simulink model "cIPC_leakyIntegrator"  (R2022a)
settings: Solver=FixedStepDiscrete  StartTime=0.0  StopTime=TMax  FixedStep=DT  RelTol=1e-3
undefined symbols (not defined in the file): DiscIntNeverNeededParam, dMdTheta, DT, K_T, Ki, optimal_azimuth_offset_rad
libraries: cstblocks x2
settings Model: Creator=jhummel  LastModifiedBy=jhummel

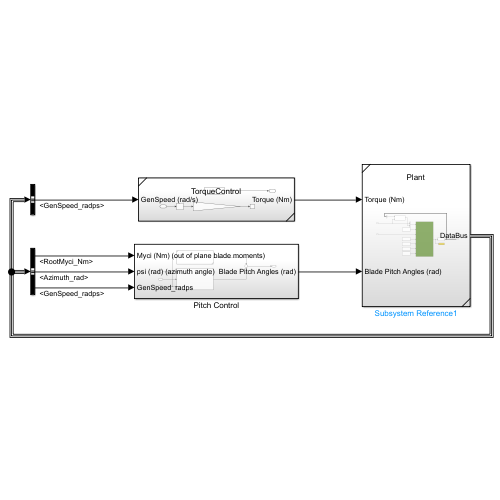
[thumbnail: Simulink's stored preview of the top-level diagram]
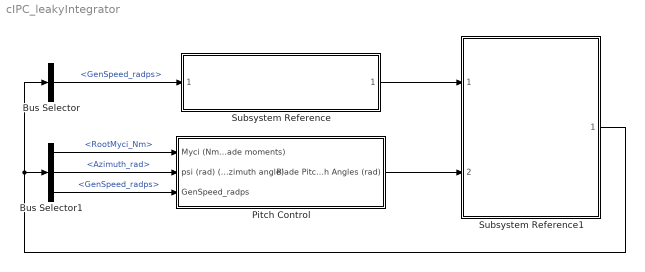
== system cIPC_leakyIntegrator ==
  Bus Selector : BusSelector  OutputSignals=GenSpeed_radps
  Bus Selector1 : BusSelector  OutputSignals=RootMyci_Nm,Azimuth_rad,GenSpeed_radps
  Pitch Control : Subsystem
  Subsystem Reference : Subsystem  ReferencedSubsystem=TorqueControl
  Subsystem Reference1 : Subsystem  ReferencedSubsystem=Plant
  wires:
  Bus Selector/1 -> Subsystem Reference/1  "<GenSpeed_radps>"
  Bus Selector1/1 -> Pitch Control/1(Myci (Nm) (out of plane blade moments))  "<RootMyci_Nm>"
  Bus Selector1/2 -> Pitch Control/2(psi (rad) (azimuth angle))  "<Azimuth_rad>"
  Bus Selector1/3 -> Pitch Control/3(GenSpeed_radps)  "<GenSpeed_radps>"
  Subsystem Reference1/1 -> Bus Selector/1, Bus Selector1/1
  Pitch Control/1(Blade Pitch Angles (rad)) -> Subsystem Reference1/2
  Subsystem Reference/1 -> Subsystem Reference1/1

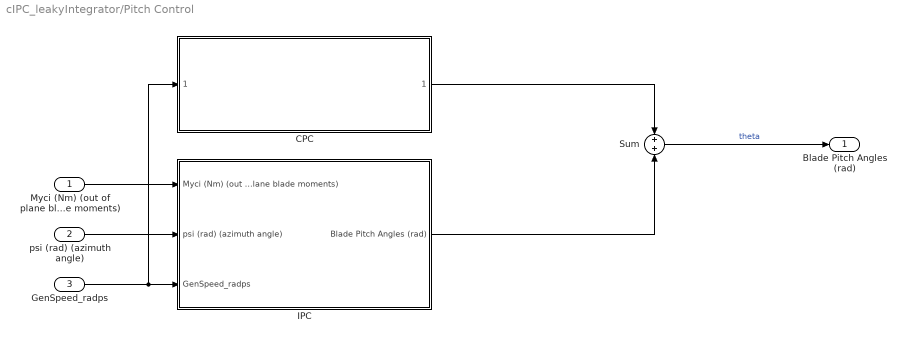
== system cIPC_leakyIntegrator/Pitch Control ==
  Myci (Nm) (out of plane blade moments) : Inport
  psi (rad) (azimuth angle) : Inport  Port=2
  GenSpeed_radps : Inport  Port=3
  CPC : Subsystem  ReferencedSubsystem=CollectivePitchControl
  IPC : Subsystem
  Sum : Sum  Inputs=+|+
  Blade Pitch Angles (rad) : Outport
  wires:
  Myci (Nm) (out of plane blade moments)/1 -> IPC/1(Myci (Nm) (out of plane blade moments))
  psi (rad) (azimuth angle)/1 -> IPC/2(psi (rad) (azimuth angle))
  GenSpeed_radps/1 -> CPC/1, IPC/3(GenSpeed_radps)
  Sum/1 -> Blade Pitch Angles (rad)/1  "theta"
  IPC/1(Blade Pitch Angles (rad)) -> Sum/2
  CPC/1 -> Sum/1

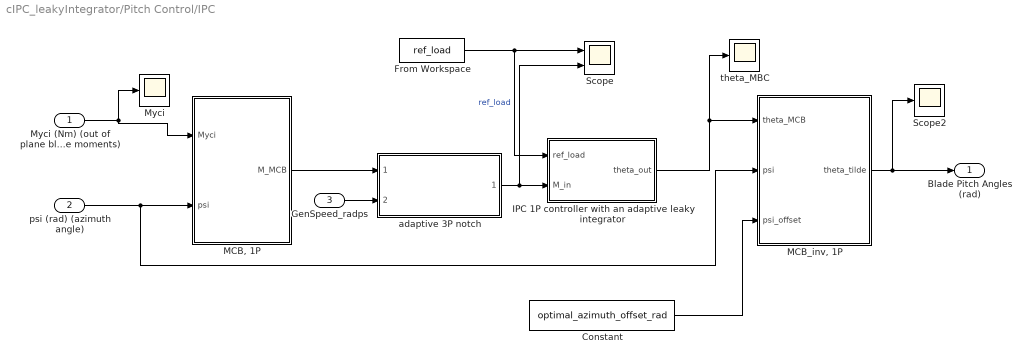
== system cIPC_leakyIntegrator/Pitch Control/IPC ==
  Myci (Nm) (out of plane blade moments) : Inport
  psi (rad) (azimuth angle) : Inport  Port=2
  GenSpeed_radps : Inport  Port=3
  Constant : Constant  Value=optimal_azimuth_offset_rad
  From Workspace : FromWorkspace  VariableName=ref_load  SampleTime=DT
  IPC 1P controller with an adaptive leaky integrator : Subsystem
  "MCB, 1P" : MATLAB Function  TreatAsAtomicUnit=on
  "MCB_inv, 1P" : MATLAB Function  TreatAsAtomicUnit=on
  Myci : Scope
  Scope : Scope  NumInputPorts=2
  Scope2 : Scope
  adaptive 3P notch : Subsystem  ReferencedSubsystem=LoadFilter
  theta_MBC : Scope
  Blade Pitch Angles (rad) : Outport
  wires:
  IPC 1P controller with an adaptive leaky integrator/1(theta_out) -> theta_MBC/1, "MCB_inv, 1P"/1(theta_MCB)
  "MCB_inv, 1P"/1(theta_tilde) -> Blade Pitch Angles (rad)/1, Scope2/1
  Myci (Nm) (out of plane blade moments)/1 -> Myci/1, "MCB, 1P"/1(Myci)
  Constant/1 -> "MCB_inv, 1P"/3(psi_offset)
  psi (rad) (azimuth angle)/1 -> "MCB_inv, 1P"/2(psi), "MCB, 1P"/2(psi)
  adaptive 3P notch/1 -> Scope/2, IPC 1P controller with an adaptive leaky integrator/2(M_in)
  GenSpeed_radps/1 -> adaptive 3P notch/2
  "MCB, 1P"/1(M_MCB) -> adaptive 3P notch/1
  From Workspace/1 -> Scope/1, IPC 1P controller with an adaptive leaky integrator/1(ref_load)  "ref_load"

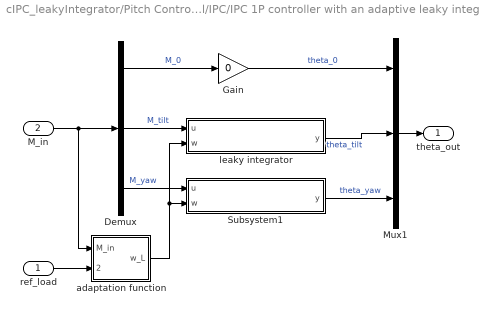
== system cIPC_leakyIntegrator/Pitch Control/IPC/IPC 1P controller with an adaptive leaky integrator ==
  ref_load : Inport
  M_in : Inport  Port=2
  Demux : Demux  Outputs=3
  Gain : Gain  Gain=0
  Mux1 : Mux  Inputs=3
  Subsystem1 : Subsystem
  adaptation function : Subsystem
  leaky integrator : Subsystem
  theta_out : Outport
  wires:
  Gain/1 -> Mux1/1  "theta_0"
  leaky integrator/1(y) -> Mux1/2  "theta_tilt"
  Demux/1 -> Gain/1  "M_0"
  Mux1/1 -> theta_out/1
  Subsystem1/1(y) -> Mux1/3  "theta_yaw"
  Demux/2 -> leaky integrator/1(u)  "M_tilt"
  M_in/1 -> adaptation function/1(M_in), Demux/1
  Demux/3 -> Subsystem1/1(u)  "M_yaw"
  ref_load/1 -> adaptation function/2(ref_load)
  adaptation function/1(w_L) -> Subsystem1/2(w), leaky integrator/2(w)

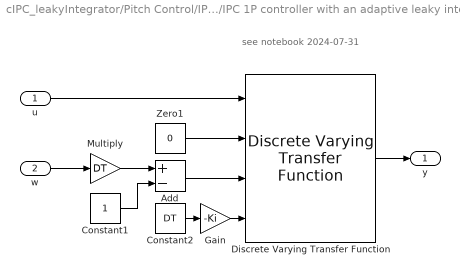
== system cIPC_leakyIntegrator/Pitch Control/IPC/IPC 1P controller with an adaptive leaky integrator/Subsystem1 ==
  note: see notebook 2024-07-31
  u : Inport
  w : Inport  Port=2
  Add : Sum  Inputs=+-
  Constant1 : Constant
  Constant2 : Constant  Value=DT
  Discrete Varying Transfer Function : cstblocks/Linear Parameter Varying/Discrete Varying Transfer Function  N=1  Ts=-1
      settings: SourceProductBaseCode=CT
  Gain : Gain  Gain=-Ki
  Multiply : Gain  Gain=DT
  Zero1 : Constant  Value=0  OutDataTypeStr=Inherit: Inherit via back propagation
  y : Outport
  wires:
  u/1 -> Discrete Varying Transfer Function/1
  Zero1/1 -> Discrete Varying Transfer Function/2
  w/1 -> Multiply/1
  Multiply/1 -> Add/1
  Constant1/1 -> Add/2
  Add/1 -> Discrete Varying Transfer Function/3
  Constant2/1 -> Gain/1
  Discrete Varying Transfer Function/1 -> y/1
  Gain/1 -> Discrete Varying Transfer Function/4

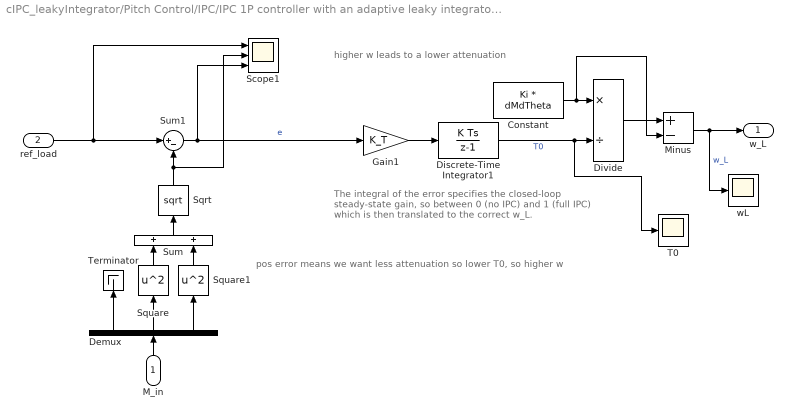
== system cIPC_leakyIntegrator/Pitch Control/IPC/IPC 1P controller with an adaptive leaky integrator/adaptation function ==
  note: pos error means we want less attenuation so lower T0, so higher w
  note: The integral of the error specifies the closed-loop steady-state gain, so between 0 (no IPC) and 1 (full IPC) which is then translated to the correct w_L.
  note: higher w leads to a lower attenuation
  M_in : Inport
  ref_load : Inport  Port=2
  Constant : Constant  Value=Ki * dMdTheta
  Demux : Demux  Outputs=3
  Discrete-Time Integrator1 : DiscreteIntegrator  InitialCondition=0.001  SampleTime=-1  LimitOutput=on  UpperSaturationLimit=1  LowerSaturationLimit=0.001  ICPrevOutput=DiscIntNeverNeededParam  ICPrevScaledInput=DiscIntNeverNeededParam
  Divide : Product  Inputs=*/
  Gain1 : Gain  Gain=K_T
  Minus : Sum  Inputs=+-
  Scope1 : Scope  NumInputPorts=3
  Sqrt : Sqrt
  Square : Math  Operator=square
  Square1 : Math  Operator=square
  Sum : Sum
  Sum1 : Sum  Inputs=|+-
  T0 : Scope
  Terminator : Terminator
  wL : Scope
  w_L : Outport
  wires:
  M_in/1 -> Demux/1
  Demux/1 -> Terminator/1
  Demux/2 -> Square/1
  Demux/3 -> Square1/1
  Square/1 -> Sum/1
  Square1/1 -> Sum/2
  Sum/1 -> Sqrt/1
  Sqrt/1 -> Scope1/2, Sum1/2
  ref_load/1 -> Scope1/1, Sum1/1
  Sum1/1 -> Scope1/3, Gain1/1  "e"
  Gain1/1 -> Discrete-Time Integrator1/1
  Discrete-Time Integrator1/1 -> T0/1, Divide/2  "T0"
  Constant/1 -> Minus/2, Divide/1
  Divide/1 -> Minus/1
  Minus/1 -> wL/1, w_L/1  "w_L"

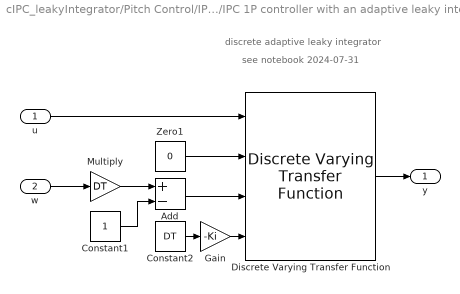
== system cIPC_leakyIntegrator/Pitch Control/IPC/IPC 1P controller with an adaptive leaky integrator/leaky integrator ==
  note: discrete adaptive leaky integrator
  note: see notebook 2024-07-31
  u : Inport
  w : Inport  Port=2
  Add : Sum  Inputs=+-
  Constant1 : Constant
  Constant2 : Constant  Value=DT
  Discrete Varying Transfer Function : cstblocks/Linear Parameter Varying/Discrete Varying Transfer Function  N=1  Ts=-1
      settings: SourceProductBaseCode=CT
  Gain : Gain  Gain=-Ki
  Multiply : Gain  Gain=DT
  Zero1 : Constant  Value=0  OutDataTypeStr=Inherit: Inherit via back propagation
  y : Outport
  wires:
  u/1 -> Discrete Varying Transfer Function/1
  Zero1/1 -> Discrete Varying Transfer Function/2
  w/1 -> Multiply/1
  Multiply/1 -> Add/1
  Constant1/1 -> Add/2
  Add/1 -> Discrete Varying Transfer Function/3
  Constant2/1 -> Gain/1
  Discrete Varying Transfer Function/1 -> y/1
  Gain/1 -> Discrete Varying Transfer Function/4

== matlab function cIPC_leakyIntegrator/Pitch Control/IPC/MCB_inv, 1P ==
  data: theta_MCB input; theta_tilde output; psi input; psi_offset input
function theta_tilde = fcn(theta_MCB, psi, psi_offset)

theta_tilde = MBC_inv(theta_MCB, psi, psi_offset, 3, 1);

end

== matlab function cIPC_leakyIntegrator/Pitch Control/IPC/MCB, 1P ==
  data: Myci input; M_MCB output; psi input
function M_MCB = fcn(Myci, psi)

% Do the coordinate transformation.
M_MCB = MBC(Myci, psi, 0, 3, 1);

end
